simulink model "cart_pole_SMC"  (R2020b)
settings: Solver=VariableStepAuto  StartTime=0.0  StopTime=10.0  RelTol=1e-3
settings Model: Creator=Taha  LastModifiedBy=Taha

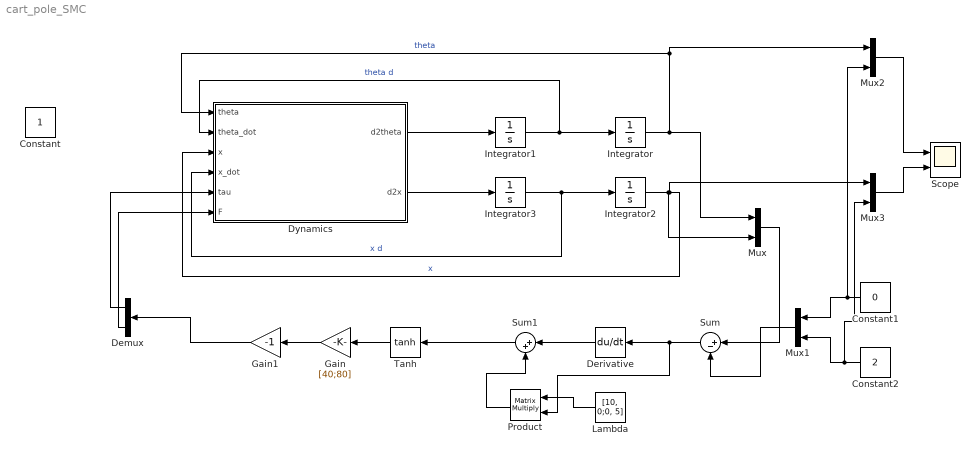
== system cart_pole_SMC ==
  Constant : Constant
  Constant1 : Constant  Value=0
  Constant2 : Constant  Value=2
  Demux : Demux  Outputs=2
  Derivative : Derivative
  Dynamics : MATLAB Function  TreatAsAtomicUnit=on
  Gain : Gain  Gain=[40;80]
  Gain1 : Gain  Gain=-1
  Integrator{,1..3} (4 alike) : Integrator
  Lambda : Constant  Value=[10, 0;0, 5]
  Mux{,1..3} (4 alike) : Mux  Inputs=2
  Product : Product  Multiplication=Matrix(*)
  Scope : Scope  NumInputPorts=2
  Sum : Sum  Inputs=|+-
  Sum1 : Sum  Inputs=|++
  Tanh : Trigonometry  Operator=tanh
  wires:
  Integrator1/1 -> Dynamics/2(theta_dot), Integrator/1  "theta d"
  Dynamics/2(d2x) -> Integrator3/1
  Dynamics/1(d2theta) -> Integrator1/1
  Integrator3/1 -> Dynamics/4(x_dot), Integrator2/1  "x d"
  Integrator2/1 -> Mux/2, Dynamics/3(x), Mux3/1  "x"
  Integrator/1 -> Mux/1, Mux2/1, Dynamics/1(theta)  "theta"
  Mux/1 -> Sum/1
  Constant1/1 -> Mux2/2, Mux1/1
  Constant2/1 -> Mux3/2, Mux1/2
  Mux1/1 -> Sum/2
  Sum/1 -> Product/2, Derivative/1
  Derivative/1 -> Sum1/1
  Lambda/1 -> Product/1
  Product/1 -> Sum1/2
  Sum1/1 -> Tanh/1
  Tanh/1 -> Gain/1
  Gain/1 -> Gain1/1
  Gain1/1 -> Demux/1
  Demux/1 -> Dynamics/5(tau)
  Demux/2 -> Dynamics/6(F)
  Mux2/1 -> Scope/1
  Mux3/1 -> Scope/2

== matlab function cart_pole_SMC/Dynamics ==
  data: theta input; theta_dot input; d2theta output; d2x output; x input; x_dot input; tau input; F input
function [d2theta,d2x ] = fcn(theta, theta_dot, x, x_dot, tau, F)
m = 1.5;
M = 6;
I = 0.6;
g = 9.81;
k = 0.75;
B = 1.2;


d2theta = (1/(I - (( m * I * cos(theta)^2) / (M+m))))...
    *(tau + g * sin(theta) + ((cos(theta) / (M + m)) * (F)) -...
    (((B * cos(theta)) / (M+m)) * (x_dot)) - (((k * cos(theta)) / (M+m)) * (x)) - ...
    (( m * I * theta_dot * sin(theta) * cos (theta)) / (M+m)));


d2x = (1 / (M+m)) * ((F)...
    - (B * x_dot)...
    -(k * x)...
    - (m * I * theta_dot * sin(theta))...
    + ((m * I * cos(theta))...
    * ( (1/(I - (( m * I * cos(theta)^2) / (M+m))))...
    *(tau + g * sin(theta) + ((cos(theta) / (M + m)) * (F)) -...
    (((B * cos(theta)) / (M+m)) * (x_dot)) - (((k * cos(theta)) / (M+m)) * (x)) - ...
    (( m * I * theta_dot * sin(theta) * cos (theta)) / (M+m))))));
